simulink model "Orbit_simu_1_R2016b"  (R2016b)
settings: Solver=VariableStepAuto  StartTime=0.0  StopTime=15000  RelTol=1e-3
libraries: aerolibconvert2 x2, aerolibgravity2 x2
settings Model: Creator=megai  LastModifiedBy=decla
settings DataIOCC: ReturnWorkspaceOutputs=on
settings SFSimCC: SimUseLocalCustomCode=on
settings RTWCC: RTWUseLocalCustomCode=on

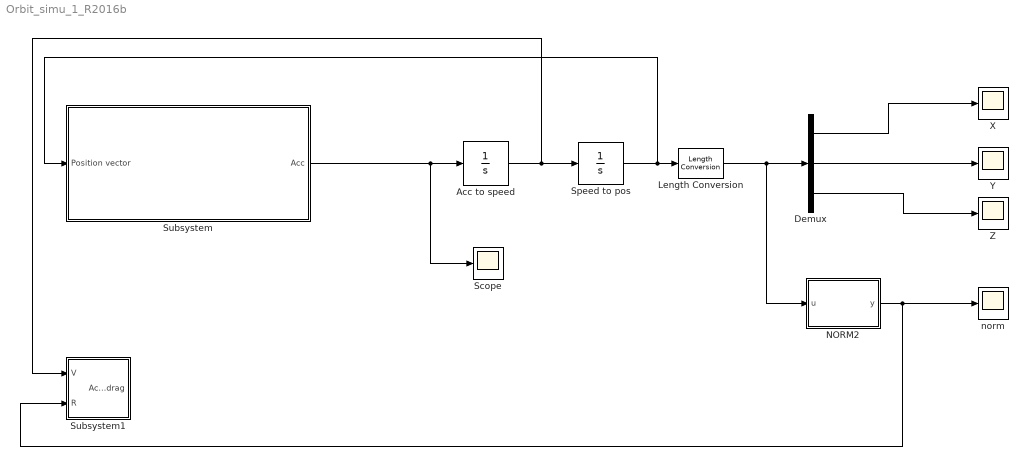
== system Orbit_simu_1_R2016b ==
  Acc to speed : Integrator  InitialCondition=[-2871.828;-5954.63;3774.64]
  Demux : Demux  Outputs=3
  Length Conversion : aerolibconvert2/Length Conversion  IU=m  OU=km
  NORM2 : MATLAB Function  TreatAsAtomicUnit=on
  Scope : Scope
  Speed to pos : Integrator  InitialCondition=[2383.89e3;2594.67e3;5906.12e3]
  Subsystem : Subsystem
  Subsystem1 : Subsystem
  X : Scope
  Y : Scope
  Z : Scope
  norm : Scope
  wires:
  Acc to speed/1 -> Subsystem1/1(V), Speed to pos/1
  Speed to pos/1 -> Length Conversion/1, Subsystem/1(Position vector)
  Subsystem/1(Acc) -> Scope/1, Acc to speed/1
  Demux/1 -> X/1
  Demux/2 -> Y/1
  Demux/3 -> Z/1
  Length Conversion/1 -> NORM2/1(u), Demux/1
  NORM2/1(y) -> Subsystem1/2(R), norm/1

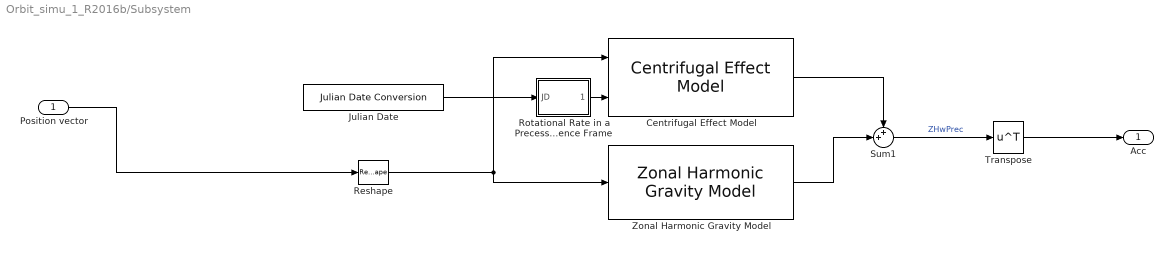
== system Orbit_simu_1_R2016b/Subsystem ==
  Position vector : Inport
  Centrifugal Effect Model : aerolibgravity2/Centrifugal Effect Model  ptype=Custom  omega=7.2921150e-005  rate_loc=on
  Julian Date : aerolibconvert2/Julian Date Conversion  year=2004  month=October  day=10  hour=12  min=21  sec=0  modflag=off  deltaT=None  errorflag=Error
  Reshape : Reshape  OutputDimensionality=Row vector (2-D)
  Rotational Rate in a Precessing Reference Frame : Subsystem
  Sum1 : Sum  Inputs=++|
  Transpose : Math  Operator=transpose  SaturateOnIntegerOverflow=on
  Zonal Harmonic Gravity Model : aerolibgravity2/Zonal Harmonic Gravity Model  units=Metric (MKS)  degree=4  action=Warning  ptype=Earth  R=6378136.3  GM=398600441500000  jvalue=[1.0826269e-03 -2.5323000e-06 -1.6204000e-06]
  Acc : Outport
  wires:
  Reshape/1 -> Centrifugal Effect Model/1, Zonal Harmonic Gravity Model/1
  Rotational Rate in a Precessing Reference Frame/1(omega) -> Centrifugal Effect Model/2
  Position vector/1 -> Reshape/1
  Julian Date/1 -> Rotational Rate in a Precessing Reference Frame/1(JD)
  Zonal Harmonic Gravity Model/1 -> Sum1/2
  Centrifugal Effect Model/1 -> Sum1/1
  Sum1/1 -> Transpose/1  "ZHwPrec"
  Transpose/1 -> Acc/1

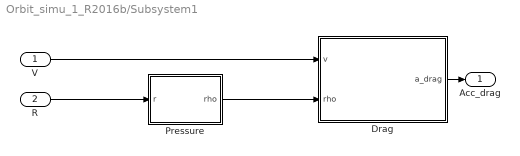
== system Orbit_simu_1_R2016b/Subsystem1 ==
  V : Inport
  R : Inport  Port=2
  Drag : MATLAB Function  TreatAsAtomicUnit=on
  Pressure : MATLAB Function  TreatAsAtomicUnit=on
  Acc_drag : Outport
  wires:
  Pressure/1(rho) -> Drag/2(rho)
  Drag/1(a_drag) -> Acc_drag/1
  V/1 -> Drag/1(v)
  R/1 -> Pressure/1(r)

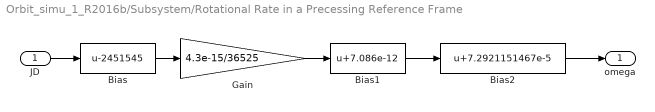
== system Orbit_simu_1_R2016b/Subsystem/Rotational Rate in a Precessing Reference Frame ==
  JD : Inport
  Bias : Bias  Bias=-2451545
  Bias1 : Bias  Bias=7.086e-12
  Bias2 : Bias  Bias=7.2921151467e-5
  Gain : Gain  Gain=4.3e-15/36525
  omega : Outport
  wires:
  JD/1 -> Bias/1
  Bias/1 -> Gain/1
  Gain/1 -> Bias1/1
  Bias1/1 -> Bias2/1
  Bias2/1 -> omega/1

== matlab function Orbit_simu_1_R2016b/Subsystem1/Drag ==
  data: v input; a_drag output; rho input
function a_drag = fcn(v, rho)
area = 100e-4;
mass = 3;
V = norm(v);
Cd = 1.05;

a_drag = -0.5*Cd*(area/mass)*rho*V^2;

== matlab function Orbit_simu_1_R2016b/Subsystem1/Pressure ==
  data: r input; rho output
function rho = fcn(r)
alt = norm(r);
A = 1.140564e-10;
B = -2.130756e-7;
C = 1.570562e-4;
D = -0.07029296;
E = -12.89844;

rho = exp(A*alt^4 + B*alt^3 + C*alt^2 + D*alt + E);

== matlab function Orbit_simu_1_R2016b/NORM2 ==
  data: u input; y output
function y = fcn(u)

y = sqrt(u(1)^2+u(2)^2+u(3)^2);
